simulink model "Book532"  (R2019b)
settings: Solver=ode4  StartTime=0.001  StopTime=20  FixedStep=0.001  RelTol=1e-3
settings Model: Creator=user  LastModifiedBy=user

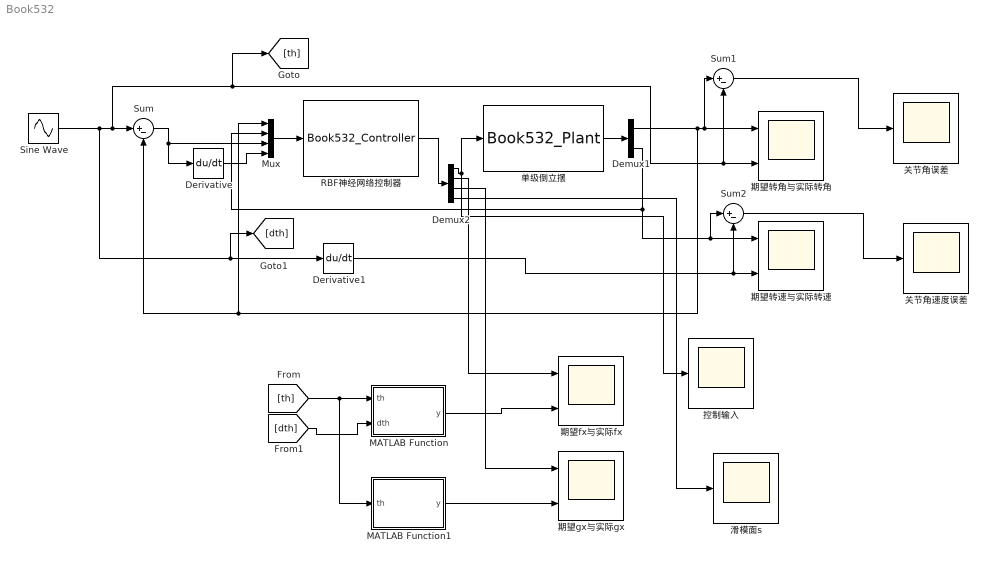
== system Book532 ==
  Demux1 : Demux  Outputs=2
  Demux2 : Demux
  Derivative : Derivative
  Derivative1 : Derivative
  MATLAB Function : MATLAB Function  TreatAsAtomicUnit=on
  MATLAB Function1 : MATLAB Function  TreatAsAtomicUnit=on
  Mux : Mux
  RBF神经网络控制器 : S-Function  FunctionName=Book532_Controller  SFunctionDeploymentMode=off  EnableBusSupport=off
  Sine Wave : Sin  Amplitude=0.1  SampleTime=0
  Sum : Sum  Inputs=|+-
  Sum1 : Sum  Inputs=|+-
  Sum2 : Sum  Inputs=|+-
  关节角误差 : Scope
  关节角速度误差 : Scope
  单级倒立摆 : S-Function  FunctionName=Book532_Plant  SFunctionDeploymentMode=off  EnableBusSupport=off
  控制输入 : Scope
  期望fx与实际fx : Scope  NumInputPorts=2
  期望gx与实际gx : Scope  NumInputPorts=2
  期望转角与实际转角 : Scope  NumInputPorts=2
  期望转速与实际转速 : Scope  NumInputPorts=2
  滑模面s : Scope
  wires:
  Sum/1 -> Mux/3, Derivative/1
  Sine Wave/1 -> [dth], Derivative1/1, [th], 期望转角与实际转角/2, Sum1/2, Sum/1
  Demux2/2 -> 期望fx与实际fx/1
  Demux1/1 -> Sum1/1, 期望转角与实际转角/1, Sum/2, Mux/1
  单级倒立摆/1 -> Demux1/1
  RBF神经网络控制器/1 -> Demux2/1
  [dth] -> MATLAB Function/2(dth)
  Mux/1 -> RBF神经网络控制器/1
  Demux1/2 -> Mux/2, Sum2/1, 期望转速与实际转速/1
  Derivative1/1 -> Sum2/2, 期望转速与实际转速/2
  MATLAB Function/1(y) -> 期望fx与实际fx/2
  [th] -> MATLAB Function1/1(th), MATLAB Function/1(th)
  Demux2/1 -> 控制输入/1, 单级倒立摆/1
  Derivative/1 -> Mux/4
  Demux2/3 -> 期望gx与实际gx/1
  MATLAB Function1/1(y) -> 期望gx与实际gx/2
  Demux2/4 -> 滑模面s/1
  Sum1/1 -> 关节角误差/1
  Sum2/1 -> 关节角速度误差/1

== matlab function Book532/MATLAB Function1 ==
  data: th input; y output
function y = fcn(th)
%#codegen
g = 9.8;
mc = 1;     %小车质量
m = 0.1;    %摆的质量
l = 0.5;
g_up = cos(th)/(mc+m);
g_down = l *(4/3 - m*(cos(th)^2)/(mc+m));
g = g_up / g_down;
y = g;

== matlab function Book532/MATLAB Function ==
  data: th input; y output; dth input
function y = fcn(th, dth)
%#codegen
g = 9.8;
mc = 1;     %小车质量
m = 0.1;    %摆的质量
l = 0.5;
f_up = g*sin(th) - m*l*dth^2*cos(th)*sin(th)/(mc+m);
f_down = l *(4/3 - m*(cos(th)^2)/(mc+m));
f = f_up / f_down;
y = f;
